simulink model "Vector_DDFS_Ex1"  (R2025a)
settings: Solver=VariableStepAuto  StartTime=0.0  StopTime=80E-6  RelTol=1e-3
InitFcn:
  | Fbits0=48; %frequency resolution
  | Abits0=16; %Sin/COS table depth is 2^Abits
  | Dbits0=18; %Sin/COS table width is 1..-Dbits
  | 
  | clk = 550e+6; % Hz
  | %clk = 275e+6; % Hz
  | 
  | % change sample rate to change SSR
  | sample_rate = 1/6600e+6; % 6.6GHz
  | sample_rate = 1/4400e+6; %
  | %sample_rate = 1/3300e+6; % 3.3GHz
  | 
  | 
  | SSR = ceil((1/sample_rate)*(1/clk));
  | Tclk = 1/clk;
  | Ts = sample_rate;
  | 
  | %SSR=128;
  | %Ts=2.5E-10; %4Gsps sample rate
  | %Tclk=SSR*Ts; %FPGA clock period
undefined symbols (not defined in the file): i, xc7vx485tffg1157
libraries: hdlBasic x4, hdlSSR x4, simulink x2, vmcUtilities x1
settings Model: Creator=admin  LastModifiedBy=robg
settings SolverCC: AlgebraicLoopSolver=TrustRegion
settings DataIOCC: ReturnWorkspaceOutputs=off
settings DebuggingCC: UnconnectedInputMsg=warning  UnconnectedOutputMsg=warning  UnconnectedLineMsg=warning  ArithmeticOperatorsInVariantConditions=warning
settings ModelReferenceCC: EnableRefExpFcnMdlSchedulingChecks=on
settings SFSimCC: SimUseLocalCustomCode=off  CustomCodeUndefinedFunction=UseInterfaceOnly
settings RTWCC: RTWUseLocalCustomCode=off  GPUComputeCapability=3.5  DLArmComputeVersion=19.05
settings CodeAppCC: StateflowObjectComments=on

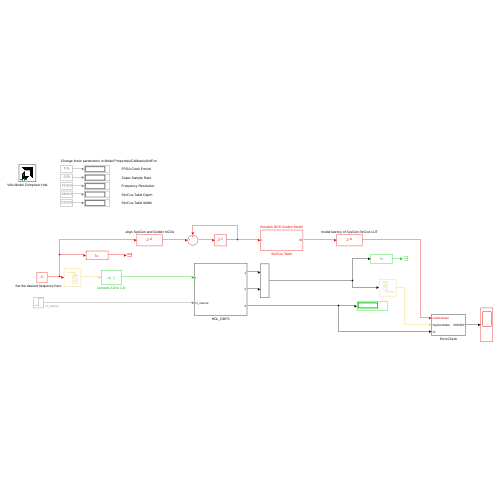
[thumbnail: Simulink's stored preview of the top-level diagram]
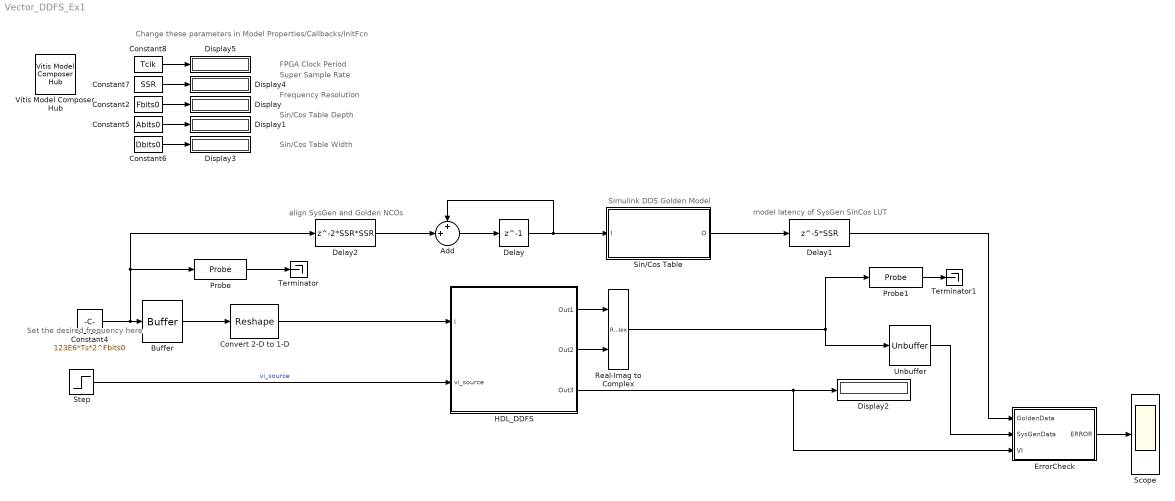
== system Vector_DDFS_Ex1 ==
  note: model latency of SysGen SinCos LUT
  note: Change these parameters in Model Properties/Callbacks/InitFcn
  note: Simulink DDS Golden Model
  note: Frequency Resolution
  note: Super Sample Rate
  note: FPGA Clock Period
  note: Set the desired frequency here
  note: Sin/Cos Table Depth
  note: Sin/Cos Table Width
  note: align SysGen and Golden NCOs
  Add : Sum  Inputs=++|  OutDataTypeStr=fixdt(1,Fbits0,0)
  Buffer : Buffer  N=SSR  OutputFrames=off
  Constant2 : Constant  Value=Fbits0  OutDataTypeStr=int32  SampleTime=-1
  Constant4 : Constant  Value=123E6*Ts*2^Fbits0  OutDataTypeStr=fixdt(1,Fbits0,0)  SampleTime=-1
  Constant5 : Constant  Value=Abits0  OutDataTypeStr=int32  SampleTime=-1
  Constant6 : Constant  Value=Dbits0  OutDataTypeStr=int32  SampleTime=-1
  Constant7 : Constant  Value=SSR  OutDataTypeStr=int32  SampleTime=-1
  Constant8 : Constant  Value=Tclk  OutDataTypeStr=double  SampleTime=-1
  Convert 2-D to 1-D : Reshape
  Delay : Delay  DelayLength=1
  Delay1 : Delay  DelayLength=5*SSR
  Delay2 : Delay  DelayLength=2*SSR*SSR
  Display{,1..5} (6 alike) : Display
  ErrorCheck : Subsystem
  HDL_DDFS : Subsystem
  Probe : Probe  ProbeWidth=off  ProbeComplexSignal=off
  Probe1 : Probe  ProbeWidth=off  ProbeComplexSignal=off
  Real-Imag to Complex : RealImagToComplex
  Scope : Scope
      settings: ActiveDisplayYMinimum=-1.25  ActiveDisplayYMaximum=1.25  DataLoggingVariableName=ScopeData2
  Sin/Cos Table : Subsystem
  Step : Step  Time=Ts
  Terminator : Terminator
  Terminator1 : Terminator
  Unbuffer : Unbuffer
  Vitis Model Composer Hub : vmcUtilities/Vitis Model Composer Hub  Tag=genX  CodeGeneration=off  SubsystemName=DDS012  StartColumn=1  NumberOfColumns=1  TargetDirectory=./code  exportDesign=off  analyzeDesign=off  validateDesignOnHw=off  ExportType=System Generator  IpVendor=xilinx.com  IpLibrary=hls  IpVersion=1.0  IpHWLanguage=Verilog  AieCompilerOptions={}  AieSimulatorOptions={}  CreateTestbench=off  TestbenchStackSize=10  RunRtlSim=off  RunCSim=off  RunAieSim=off  enableSimulationTimeout=on  enableGraphIterations=on  AieSimTimeout=50000  AieGraphIterations=-1  RunAieSimProfiling=off  LaunchVitisAnalyzer=off  PlotOutput=off  RunX86Sim=off  X86SimTimeout=10  GenHwImage=off  GenLibadfXo=off  GenHwValidationCode=off  PlatformType=Not Specified  HwSystemType=Baremetal  HwValidationTarget=hw  ProjDevice=xc7vx485tffg1157-1  SamplePeriod=-1  ClockFrequency=200  DataPathParallelism=1  xilinxfamily=kintexuplus  part=xcku9p  speed=-1-e  package=ffve900  directory=./netlist  testbench=off  incr_netlist=off  synthesis_tool=Vivado  clock_wrapper=Clock Enables  dbl_ovrd=According to Block Masks  dcm_input_clock_period=10  sysclk_period=(1e+9)/clk  simulink_period=1/clk  eval_field=0  LogFileName=''  NThreads=4
  wires:
  Constant4/1 -> Buffer/1, Delay2/1, Probe/1
  Buffer/1 -> Convert 2-D to 1-D/1
  Add/1 -> Delay/1
  Constant2/1 -> Display/1
  Constant5/1 -> Display1/1
  Constant6/1 -> Display3/1
  Probe/1 -> Terminator/1
  Constant7/1 -> Display4/1
  Probe1/1 -> Terminator1/1
  Constant8/1 -> Display5/1
  Sin/Cos Table/1(O) -> Delay1/1
  Real-Imag to Complex/1 -> Unbuffer/1, Probe1/1
  Unbuffer/1 -> ErrorCheck/2(SysGenData)
  ErrorCheck/1(ERROR) -> Scope/1
  Delay1/1 -> ErrorCheck/1(GoldenData)
  Delay/1 -> Sin/Cos Table/1(I), Add/1
  Delay2/1 -> Add/2
  HDL_DDFS/3(Out3) -> ErrorCheck/3(VI), Display2/1
  Convert 2-D to 1-D/1 -> HDL_DDFS/1(I)
  Step/1 -> HDL_DDFS/2(vi_source)  "vi_source"
  HDL_DDFS/1(Out1) -> Real-Imag to Complex/1
  HDL_DDFS/2(Out2) -> Real-Imag to Complex/2

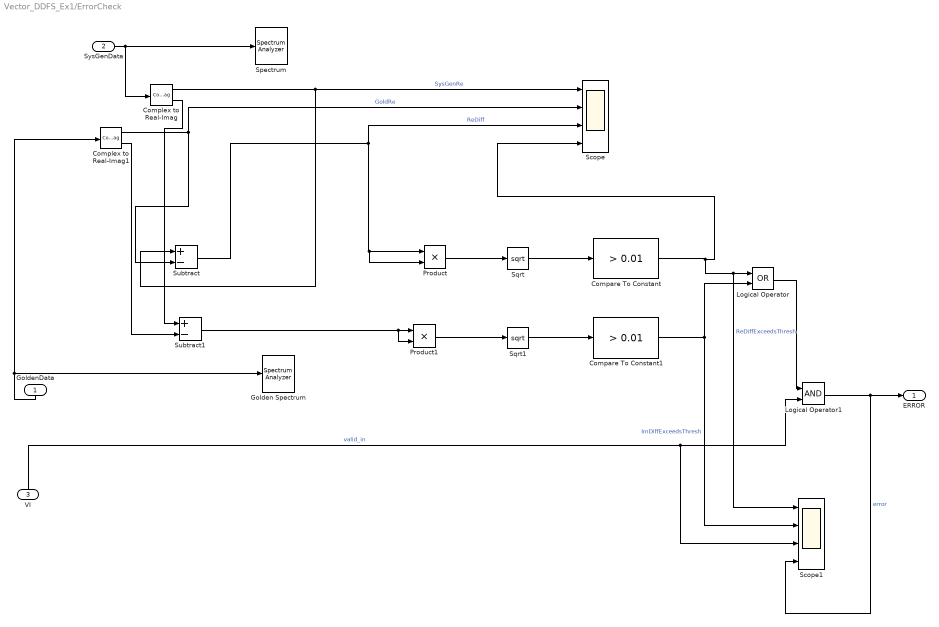
== system Vector_DDFS_Ex1/ErrorCheck ==
  GoldenData : Inport
  SysGenData : Inport  Port=2
  VI : Inport  Port=3
  Compare To Constant : simulink/Logic and Bit Operations/Compare To Constant  relop=>  const=0.01  OutDataTypeStr=boolean
  Compare To Constant1 : simulink/Logic and Bit Operations/Compare To Constant  relop=>  const=0.01  OutDataTypeStr=boolean
  Complex to Real-Imag : ComplexToRealImag
  Complex to Real-Imag1 : ComplexToRealImag
  Golden Spectrum : SpectrumAnalyzer  Method=Welch  AxesScaling=Manual  WindowLength=10000  AveragingMethod=Exponential  ChannelNames="[\"\"]"  AllowFFTLengthLessThanSamplesPerUpdate=on  DefaultConfigurationName=spbscopes.SpectrumAnalyzerBlockCfg
  Logical Operator : Logic  Operator=OR  AllPortsSameDT=off  OutDataTypeStr=boolean
  Logical Operator1 : Logic  AllPortsSameDT=off  OutDataTypeStr=boolean
  Product : Product
  Product1 : Product
  Scope : Scope  NumInputPorts=4
      settings: ActiveDisplayYMinimum=-1.2494  ActiveDisplayYMaximum=1.2447
  Scope1 : Scope  NumInputPorts=4
      settings: ActiveDisplayYMinimum=-0.125  ActiveDisplayYMaximum=1.125
  Spectrum : SpectrumAnalyzer  Method=Welch  AxesScaling=Manual  WindowLength=10000  AveragingMethod=Exponential  ChannelNames="[\"\"]"  AllowFFTLengthLessThanSamplesPerUpdate=on  DefaultConfigurationName=spbscopes.SpectrumAnalyzerBlockCfg
  Sqrt : Sqrt
  Sqrt1 : Sqrt
  Subtract : Sum  Inputs=+-
  Subtract1 : Sum  Inputs=+-
  ERROR : Outport
  wires:
  Complex to Real-Imag/1 -> Subtract/1, Scope/1  "SysGenRe"
  Complex to Real-Imag1/1 -> Scope/2, Subtract/2  "GoldRe"
  Subtract/1 -> Scope/3, Product/2, Product/1  "ReDiff"
  GoldenData/1 -> Golden Spectrum/1, Complex to Real-Imag1/1
  SysGenData/1 -> Complex to Real-Imag/1, Spectrum/1
  Product/1 -> Sqrt/1
  Sqrt/1 -> Compare To Constant/1
  Logical Operator/1 -> Logical Operator1/1
  Compare To Constant/1 -> Scope/4, Scope1/1, Logical Operator/1  "ReDiffExceedsThresh"
  Subtract1/1 -> Product1/2, Product1/1
  Product1/1 -> Sqrt1/1
  Sqrt1/1 -> Compare To Constant1/1
  Complex to Real-Imag/2 -> Subtract1/1
  Complex to Real-Imag1/2 -> Subtract1/2
  Logical Operator1/1 -> Scope1/4, ERROR/1  "error"
  VI/1 -> Scope1/3, Logical Operator1/2  "valid_in"
  Compare To Constant1/1 -> Scope1/2, Logical Operator/2  "ImDiffExceedsThresh"

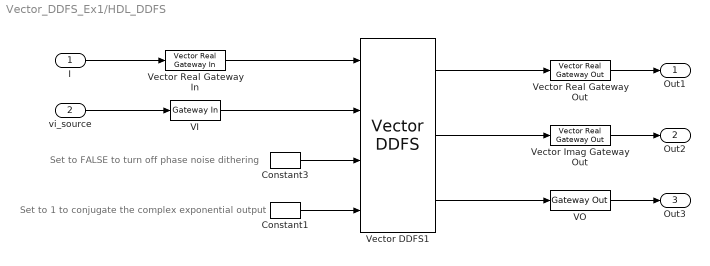
== system Vector_DDFS_Ex1/HDL_DDFS ==
  note: Set to 1 to conjugate the complex exponential output
  note: Set to FALSE to turn off phase noise dithering
  I : Inport
  vi_source : Inport  Port=2
  Constant1 : hdlBasic/Constant  const=0  gui_display_data_type=Fixed-point  arith_type=Unsigned  n_bits=1  bin_pt=0  preci_type=Single  exp_width=8  frac_width=24  explicit_period=on  period=Tclk  XmcBlockStatus=1  maskContainerNames=tabcontainer1  block_type=constant  block_config=sysgen:Constant_config
  Constant3 : hdlBasic/Constant  const=1  gui_display_data_type=Boolean  arith_type=Boolean  n_bits=1  bin_pt=0  preci_type=Single  exp_width=8  frac_width=24  explicit_period=on  period=Tclk  XmcBlockStatus=1  maskContainerNames=tabcontainer1  block_type=constant  block_config=sysgen:Constant_config
  VI : hdlBasic/Gateway In  gui_display_data_type=Boolean  arith_type=Boolean  n_bits=48  bin_pt=0  preci_type=Single  exp_width=8  frac_width=24  rows=1  columns=1  quantization="Round  (unbiased: +/- Inf)"  overflow=Saturate  period=Tclk  UseAsADC=off  ADCChannel='1'  interface=None  automatic_assignment=on  address_offset=hex2dec('00')  intf_name=''  intf_description=''  default_value=0  timing_constraint=None  locs_specified=off  LOCs={}  io_standard={}  inherit_from_input=off  hdl_port=on  XmcBlockStatus=1  maskContainerNames=group4  block_type=gatewayin  block_config=sysgen:gateway_in_config  block_width_w=590  block_height_w=620  block_width=640  block_height=850
  VO : hdlBasic/Gateway Out  inherit_from_input=off  bool_to_boolean=off  hdl_port=on  rows=1  columns=1  UseAsDAC=off  DACChannel='1'  interface=None  automatic_assignment=on  address_offset=hex2dec('00')  intf_name=''  intf_description=''  timing_constraint=None  locs_specified=off  LOCs={}  io_standard={}  XmcBlockStatus=1  maskContainerNames=group4  block_type=gatewayout  block_config=sysgen:gateway_out_config  block_width_w=590  block_height_w=620  block_width=620  block_height=750
  Vector DDFS1 : hdlSSR/Vector DDFS  sg_ssr=SSR  Fbits=Fbits0  Abits=Abits0  Dbits=Dbits0  block_type=ddfs_ssr  XmcBlockStatus=1  sg_ssr_prev=8  maskContainerNames=group1
  Vector Imag Gateway Out : hdlSSR/Vector Real Gateway Out  inherit_from_input=off  hdl_port=on  sg_ssr=SSR  rows=1  columns=1  UseAsDAC=off  DACChannel='1'  interface=None  automatic_assignment=on  address_offset=hex2dec('00')  intf_name=''  intf_description=''  timing_constraint=None  locs_specified=off  LOCs={}  io_standard={}  block_type=realgatewayout_ssr  XmcBlockStatus=1  sg_ssr_prev=32  maskContainerNames=group4  block_width_w=590  block_height_w=620  block_width=620  block_height=750
  Vector Real Gateway In : hdlSSR/Vector Real Gateway In  gui_display_data_type=Fixed-point  arith_type=Signed (2's comp)  n_bits=Fbits0  bin_pt=0  preci_type=Single  exp_width=8  frac_width=24  quantization=Truncate  overflow=Wrap  period=Tclk  sg_ssr=SSR  UseAsADC=off  ADCChannel='1'  interface=None  automatic_assignment=on  address_offset=hex2dec('00')  intf_name=''  intf_description=''  default_value=0  timing_constraint=None  locs_specified=off  LOCs={}  io_standard={}  inherit_from_input=off  hdl_port=on  interface_prev=1  block_type=realgatewayin_ssr  XmcBlockStatus=1  sg_ssr_prev=8  maskContainerNames=group4  block_width_w=590  block_height_w=670  block_width=640  block_height=850
  Vector Real Gateway Out : hdlSSR/Vector Real Gateway Out  inherit_from_input=off  hdl_port=on  sg_ssr=SSR  rows=1  columns=1  UseAsDAC=off  DACChannel='1'  interface=None  automatic_assignment=on  address_offset=hex2dec('00')  intf_name=''  intf_description=''  timing_constraint=None  locs_specified=off  LOCs={}  io_standard={}  block_type=realgatewayout_ssr  XmcBlockStatus=1  sg_ssr_prev=32  maskContainerNames=group4  block_width_w=590  block_height_w=620  block_width=620  block_height=750
  Out1 : Outport
  Out2 : Outport  Port=2
  Out3 : Outport  Port=3
  wires:
  Vector DDFS1/1 -> Vector Real Gateway Out/1
  VI/1 -> Vector DDFS1/2
  Vector DDFS1/3 -> VO/1
  VO/1 -> Out3/1
  Vector Real Gateway In/1 -> Vector DDFS1/1
  vi_source/1 -> VI/1
  Vector DDFS1/2 -> Vector Imag Gateway Out/1
  Vector Real Gateway Out/1 -> Out1/1
  Constant3/1 -> Vector DDFS1/3
  Constant1/1 -> Vector DDFS1/4
  I/1 -> Vector Real Gateway In/1
  Vector Imag Gateway Out/1 -> Out2/1

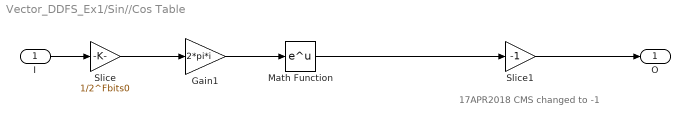
== system Vector_DDFS_Ex1/Sin//Cos Table ==
  note: 17APR2018 CMS changed to -1
  I : Inport
  Gain1 : Gain  Gain=2*pi*i  OutDataTypeStr=double
  Math Function : Math  SignedPower=on
  Slice : Gain  Gain=1/2^Fbits0  OutDataTypeStr=fixdt(1,Abits0,Abits0)
  Slice1 : Gain  Gain=-1  OutDataTypeStr=fixdt(1,Dbits0+2,Dbits0)
  O : Outport
  wires:
  Slice/1 -> Gain1/1
  Gain1/1 -> Math Function/1
  Math Function/1 -> Slice1/1
  I/1 -> Slice/1
  Slice1/1 -> O/1
